simulink model "tests_2"  (R2020b)
settings: Solver=ode45  StartTime=0.0  StopTime=10  MaxStep=1e-3  RelTol=1e-3
settings Model: Creator=kika  LastModifiedBy=kika

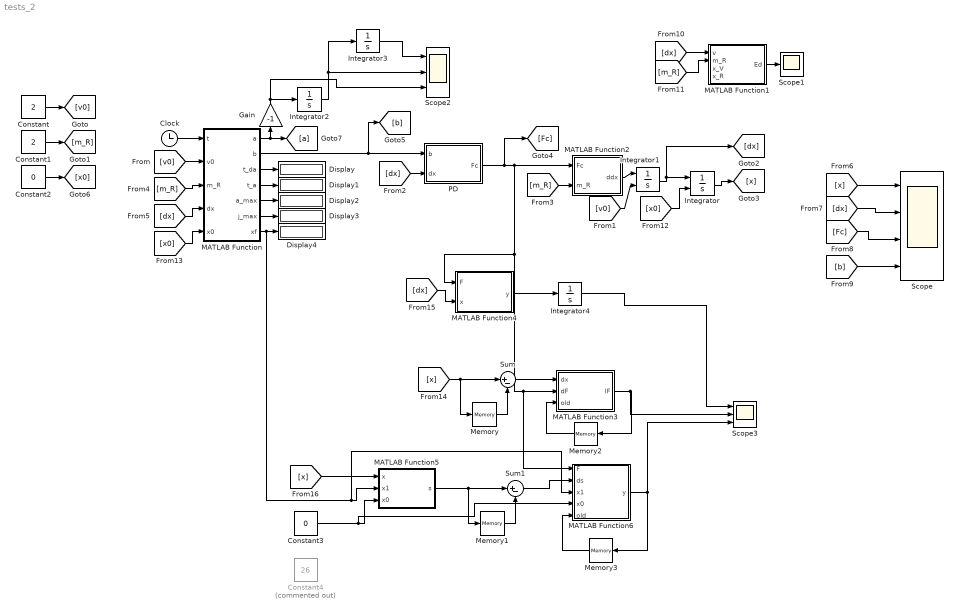
== system tests_2 ==
  Clock : Clock
  Constant : Constant  Value=2
  Constant1 : Constant  Value=2
  Constant2 : Constant  Value=0
  Constant3 : Constant  Value=0
  Constant4 : Constant  Commented=on  Value=26
  Display{,1..4} (5 alike) : Display
  Gain : Gain  Gain=-1
  Integrator : Integrator  InitialConditionSource=external
  Integrator1 : Integrator  InitialConditionSource=external  InitialCondition=1
  Integrator2 : Integrator  InitialCondition=1
  Integrator3 : Integrator
  Integrator4 : Integrator
  MATLAB Function : MATLAB Function  TreatAsAtomicUnit=on
  MATLAB Function1 : MATLAB Function  TreatAsAtomicUnit=on
  MATLAB Function2 : MATLAB Function  TreatAsAtomicUnit=on
  MATLAB Function3 : MATLAB Function  TreatAsAtomicUnit=on
  MATLAB Function4 : MATLAB Function  TreatAsAtomicUnit=on
  MATLAB Function5 : MATLAB Function  TreatAsAtomicUnit=on
  MATLAB Function6 : MATLAB Function  TreatAsAtomicUnit=on
  Memory{,1..3} (4 alike) : Memory
  PD : MATLAB Function  TreatAsAtomicUnit=on
  Scope : Scope  NumInputPorts=4
  Scope1 : Scope
  Scope2 : Scope  NumInputPorts=3
  Scope3 : Scope  NumInputPorts=3
  Sum : Sum  Inputs=|+-
  Sum1 : Sum  Inputs=|+-
  wires:
  Clock/1 -> MATLAB Function/1(t)
  Constant/1 -> [v0]
  [v0] -> MATLAB Function/2(v0)
  Constant1/1 -> [m_R]
  MATLAB Function2/1(ddx) -> Integrator1/1
  PD/1(Fc) -> MATLAB Function2/1(Fc), MATLAB Function6/1(F), MATLAB Function3/2(dF), MATLAB Function4/1(F), [Fc]
  [v0] -> Integrator1/2
  Integrator/1 -> [x]
  [dx] -> PD/2(dx)
  [m_R] -> MATLAB Function2/2(m_R)
  [m_R] -> MATLAB Function/3(m_R)
  [dx] -> MATLAB Function/4(dx)
  [x] -> Scope/1
  [dx] -> Scope/2
  [Fc] -> Scope/3
  MATLAB Function/2(b) -> [b], PD/1(b)
  [b] -> Scope/4
  [dx] -> MATLAB Function1/1(v)
  [m_R] -> MATLAB Function1/2(m_R)
  MATLAB Function1/1(Ed) -> Scope1/1
  Gain/1 -> Integrator2/1, Scope2/3
  MATLAB Function/3(t_da) -> Display/1
  MATLAB Function/4(t_a) -> Display1/1
  MATLAB Function/5(a_max) -> Display2/1
  MATLAB Function/6(j_max) -> Display3/1
  [x0] -> Integrator/2
  Constant2/1 -> [x0]
  [x0] -> MATLAB Function/5(x0)
  Integrator2/1 -> Integrator3/1, Scope2/2
  Integrator3/1 -> Scope2/1
  MATLAB Function/1(a) -> [a], Gain/1
  [x] -> Memory/1, Sum/1
  Memory/1 -> Sum/2
  Sum/1 -> MATLAB Function3/1(dx)
  Memory2/1 -> MATLAB Function3/3(old)
  MATLAB Function3/1(IF) -> Scope3/2, Memory2/1
  Integrator4/1 -> Scope3/1
  MATLAB Function4/1(y) -> Integrator4/1
  Integrator1/1 -> [dx], Integrator/1
  [dx] -> MATLAB Function4/2(x)
  Memory1/1 -> Sum1/2
  MATLAB Function5/1(s) -> Memory1/1, Sum1/1
  [x] -> MATLAB Function5/1(x)
  Constant3/1 -> MATLAB Function6/4(x0), MATLAB Function5/3(x0)
  MATLAB Function/7(xf) -> MATLAB Function6/3(x1), MATLAB Function5/2(x1), Display4/1
  MATLAB Function6/1(y) -> Scope3/3, Memory3/1
  Memory3/1 -> MATLAB Function6/5(old)
  Sum1/1 -> MATLAB Function6/2(ds)

== matlab function tests_2/MATLAB Function1 ==
  data: v input; Ed output; m_R input; x_V input; x_R input
function Ed = fcn(v, m_R, x_V, x_R)

%     e = x_V - x_R;
    Ed = 0.5 * m_R * v^2;
%     Es = 0.5 * k * e^2;

== matlab function tests_2/MATLAB Function ==
  data: a output; t input; b output; v0 input; m_R input; dx input; t_da output; t_a output; a_max output; j_max output; xf output; x0 input
function [a,b, t_da, t_a, a_max, j_max, xf] = fcn(t, v0, m_R, dx, x0)


    F_max = 3.3;
    a_max = F_max / m_R;
    
    t_da = abs(v0) / a_max;
    
    j_max = 10;
    
    t_a = a_max / j_max;
    t_da = abs(v0) / a_max + t_a;
    
    xf = v0^2/ (2*a_max);
    xf = xf + xf * t_a / t_da;
% $    xf = x0 + v0 * t_da - 0.5 * a_max * t_da^2 + 0.1667 * j_max * t_da^3;
    
    a = 0;
    if t <= t_a
        a = sign(v0) * j_max * t;
    elseif t <= (t_da - t_a)
        a = sign(v0) * a_max;
    elseif t <= t_da
        a = sign(v0) * (j_max * t_da - j_max * t);
    end
    b = m_R * a / dx;

== matlab function tests_2/PD ==
  data: b input; Fc output; dx input
function Fc = fcn(b, dx)

Fc = - b * dx;

== matlab function tests_2/MATLAB Function2 ==
  data: Fc input; ddx output; m_R input
function ddx = robot(Fc, m_R)

ddx = 1/m_R * Fc;

== matlab function tests_2/MATLAB Function3 ==
  data: dx input; IF output; dF input; old input
function IF = fcn(dx, dF, old)

IF = old + dF * dx;

== matlab function tests_2/MATLAB Function4 ==
  data: F input; y output; x input
function y = fcn(F, x)

y = F * x;

== matlab function tests_2/MATLAB Function5 ==
  data: x input; s output; x1 input; x0 input
function s = fcn(x, x1, x0)

s = (x - x0) / (x1 - x0);

== matlab function tests_2/MATLAB Function6 ==
  data: F input; y output; ds input; x1 input; x0 input; old input
function y = fcn(F, ds, x1, x0, old)

y = old + F * (x1 - x0) * ds;
